simulink model "pid_wwh"  (R2018a)
settings: Solver=ode45  StartTime=0.0  StopTime=10.0  RelTol=1e-3  EnableMultiTasking=on
PreLoadFcn:
  | Ts = 0.2;
undefined symbols (not defined in the file or in its folder): Kd, Ki, Kp
settings Model: Creator=nicholas  LastModifiedBy=Will
settings DataIOCC: LimitDataPoints=on  SaveFormat=Array  SignalLoggingName=sigsOut
settings OptimizationCC: ExpressionDepthLimit=2147483647  InitFltsAndDblsToZero=on  LifeSpan=inf
settings DebuggingCC: SaveWithParameterizedLinksMsg=none  UnderspecifiedInitializationDetection=Classic  MergeDetectMultiDrivingBlocksExec=none  SignalResolutionControl=TryResolveAllWithWarning  MultiTaskDSMMsg=warning  MultiTaskCondExecSysMsg=none  ParameterPrecisionLossMsg=none  FcnCallInpInsideContextMsg=warning  AllowSymbolicDim=off  StateNameClashWarn=warning  SFUnexpectedBacktrackingDiag=warning  SFNoUnconditionalDefaultTransitionDiag=warning  SFExecutionAtInitializationDiag=none
settings HardwareCC: ProdBitPerPointer=32  ProdBitPerSizeT=32  ProdBitPerPtrDiffT=32  ProdLargestAtomicFloat=None  ProdIntDivRoundTo=Undefined  ProdEndianess=Unspecified  ProdWordSize=32  ProdHWDeviceType=32-bit Generic  TargetUnknown=on
settings ModelReferenceCC: PropagateSignalLabelsOutOfModel=off
settings CodeAppCC: StateflowObjectComments=on
settings GRTTargetCC: TargetFcnLib=ansi_tfl_tmw.mat  TargetLangStandard=C89/C90 (ANSI)  GeneratePreprocessorConditionals=Disable all  CombineOutputUpdateFcns=off  GRTInterface=on
settings ConfigComp: CovMetricSettings=dw  CovHtmlReporting=on  CovSaveCumulativeToWorkspaceVar=on  CovSaveSingleToWorkspaceVar=on  CovExternalEMLEnable=off  CovSFcnEnable=off

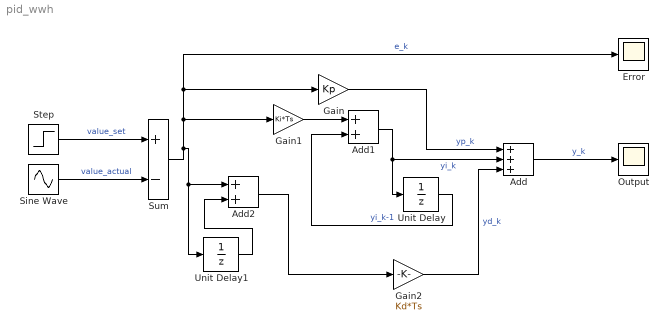
== system pid_wwh ==
  Add : Sum  Inputs=+++
  Add1 : Sum
  Add2 : Sum
  Error : Scope
  Gain : Gain  Gain=Kp
  Gain1 : Gain  Gain=Ki*Ts
  Gain2 : Gain  Gain=Kd*Ts
  Output : Scope
  Sine Wave : Sin  SampleTime=Ts
  Step : Step  SampleTime=Ts
  Sum : Sum  Inputs=+-  SaturateOnIntegerOverflow=on  InputSameDT=on  OutDataTypeStr=Inherit: Same as first input
  Unit Delay : UnitDelay  SampleTime=-1
  Unit Delay1 : UnitDelay  SampleTime=-1
  wires:
  Add/1 -> Output/1  "y_k"
  Step/1 -> Sum/1  "value_set"
  Sine Wave/1 -> Sum/2  "value_actual"
  Gain/1 -> Add/1  "yp_k"
  Gain1/1 -> Add1/1
  Add1/1 -> Add/2, Unit Delay/1  "yi_k"
  Unit Delay/1 -> Add1/2  "yi_k-1"
  Unit Delay1/1 -> Add2/2
  Add2/1 -> Gain2/1
  Gain2/1 -> Add/3  "yd_k"
  Sum/1 -> Unit Delay1/1, Add2/1, Error/1, Gain/1, Gain1/1  "e_k"
